simulink model "Friction_simulation"  (R2017b)
settings: Solver=FixedStepAuto  StartTime=0.0  StopTime=24  FixedStep=0.0005  MaxStep=0.0005  MinStep=0.0005  RelTol=1e-3
settings Model: Creator=zkt  LastModifiedBy=zkt

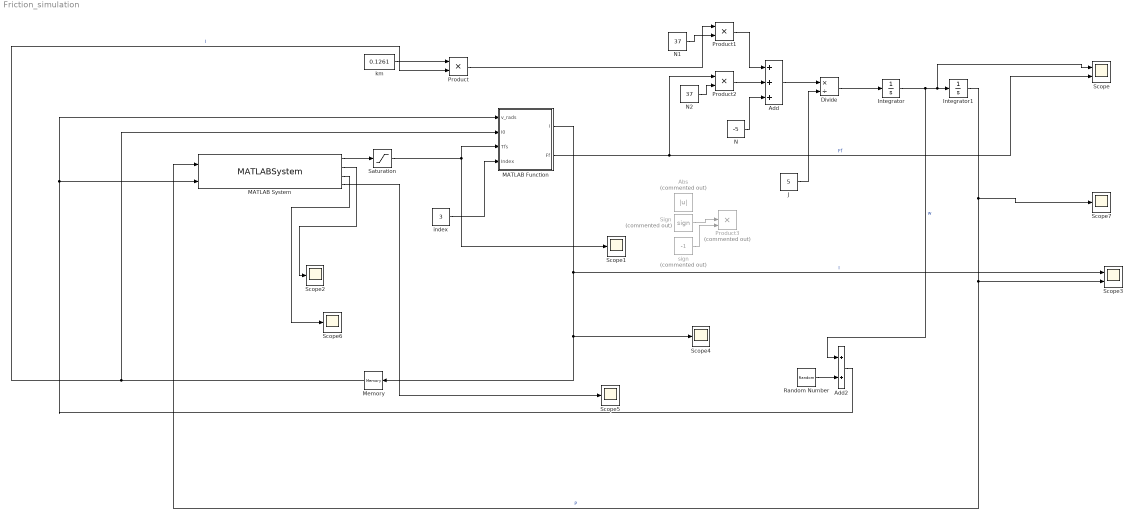
== system Friction_simulation ==
  Abs : Abs  Commented=on
  Add : Sum  Inputs=+++
  Add2 : Sum
  Divide : Product  Inputs=*/
  Integrator : Integrator
  Integrator1 : Integrator
  J : Constant  Value=5  OutDataTypeStr=double
  MATLAB Function : MATLAB Function  TreatAsAtomicUnit=on
  MATLAB System : MATLABSystem  System=Friction_simulation_control  SimulateUsing=Code generation
      mask Type: Friction_simulation_control
      mask Display:
      | disp('Friction_simulation_control');
      | port_label('input',1,'actuator_position');
      | port_label('input',2,'actuator_velocity');
      | port_label('output',1,'target_torque');
      | port_label('output',2,'random_w');
      | port_label('output',3,'random_I');
      | port_label('output',4,'simu_step');
  Memory : Memory
  N : Constant  Value=-5  OutDataTypeStr=double
  N1 : Constant  Value=37  OutDataTypeStr=double
  N2 : Constant  Value=37  OutDataTypeStr=double
  Product : Product
  Product1 : Product
  Product2 : Product
  Product3 : Product  Commented=on  Inputs=3
  Random Number : RandomNumber  Variance=0.01  SampleTime=0.0005
  Saturation : Saturate  UpperLimit=100  LowerLimit=-100
  Scope : Scope  NumInputPorts=2
  Scope{1..2,4..7} (6 alike) : Scope
  Scope3 : Scope  NumInputPorts=2
  Sign : Signum  Commented=on
  "index " : Constant  Value=3  OutDataTypeStr=int16
  km : Constant  Value=0.1261  OutDataTypeStr=double
  sign : Constant  Commented=on  Value=-1  OutDataTypeStr=double
  wires:
  km/1 -> Product/1
  Add/1 -> Divide/1
  Product/1 -> Product1/1
  "index "/1 -> MATLAB Function/4(Index)
  MATLAB Function/1(I) -> Memory/1, Scope4/1, Scope3/1  "I"
  J/1 -> Divide/2
  Divide/1 -> Integrator/1
  MATLAB System/2 -> Scope2/1
  N/1 -> Add/3
  MATLAB System/1 -> Saturation/1
  N1/1 -> Product1/2
  Product1/1 -> Add/1
  N2/1 -> Product2/2
  Product2/1 -> Add/2
  Integrator1/1 -> Scope7/1, Scope3/2, MATLAB System/1  "P"
  Saturation/1 -> MATLAB Function/3(Tfs), Scope1/1
  MATLAB System/4 -> Scope5/1
  MATLAB Function/2(Ff) -> Product2/1, Scope/2  "Ff"
  Sign/1 -> Product3/2
  sign/1 -> Product3/3
  MATLAB System/3 -> Scope6/1
  Random Number/1 -> Add2/2
  Integrator/1 -> Add2/1, Scope/1, Integrator1/1  "w"
  Memory/1 -> MATLAB Function/2(I0), Product/2  "I"
  Add2/1 -> MATLAB System/2, MATLAB Function/1(v_rads)

== matlab function Friction_simulation/MATLAB Function ==
  data: v_rads input; I output; I0 input; Tfs input; Index input; Ff output
function [I,Ff] = GetCurrent(v_rads,I0,Tfs,Index) %v:rad/s I:A %Tfs:NM output_torque 
    if Index ==3 || Index ==4   %三维模型
%         sigmoid_zoom = 2000;
        Km = 2.9/23;  %0.1261
        N=37; %减速比
        Te=I0*Km; %Te电扭矩 
%         v_rads_sign_current = sign(I0)*abs(v_rads);
        if v_rads >0 
            Ff = f_PO(v_rads,Te,Index);
        else
            Ff = f_NE(v_rads,Te,Index);
        end      
%         Ff = Ff*0.5;
        I=(Tfs-N*Ff)/(N*Km);
    elseif Index == 1    %旧模型
%         start_average =  1.39;
        Km1 = 2.9/23;
        N1=50;
        Te=I0*Km1; %Te电扭矩
%         v_rads_sign_current = sign(I0)*abs(v_rads);
        if v_rads > 0    
            Ff = f_PO_xiebo(v_rads,Te,Index);
        else 
            Ff = f_NE_xiebo(v_rads,Te,Index);
        end
%         Ff = Ff*0.5;
        I=(Tfs-N1*Ff)/(N1*Km1);
    else
        Ff =0;
        I= 0;
    end
end


function [z]= f_PO_xiebo(x,y,Index)
    ac = -0.5709;    
    as = -0.3521;  
    fc = 0.1078 ;
    fs = 0.1346; %adjust
    sigma = 0.009376;
    vs = 0.08399;
    z = -(fc+ac*y)-(fs+as*y-fc-ac*y)*exp(-x/vs)-sigma*x;
end
function [z]= f_NE_xiebo(x,y,Index)
    ac = -0.5873;    
    as = -0.332;  
    fc = 0.1144;
    fs = 0.1387; %adjust
    sigma =  0.0108;
    vs = 0.09723;
    z = fc-ac*y+(fs-as*y-fc+ac*y)*exp(x/vs)-sigma*x;
end
function [z]= f_PO(x,y,Index) 
%result
%        ac 常系数，表征电扭矩对库伦摩擦力矩的影响
%        as 常系数，表征电扭矩对静摩擦力矩的影响
%        fc 库伦摩擦力矩常数项
%        fs 静摩擦力矩常数项
%        sigma 粘滞摩擦系数
%        vs 临界Stribeck速度
%        x 速度rad/s
%        y 电扭矩NM=I*km
%        km=0.1261
% %PO:z1=f(x1,y1)
% General model:
%      f(x,y) = -(fc+ac*y)-(fs+as*y-fc-ac*y)*exp(-x/vs)-sigma*x
% Coefficients (with 95% confidence bounds):
%        ac =      0.1282  (0.1255, 0.131)
%        as =     0.08165  (0.06208, 0.1012)
%        fc =      0.1958  (0.1925, 0.1992)
%        fs =      0.3001  (0.2872, 0.313)
%        sigma =     0.02891  (0.02746, 0.03036)
%        vs =      0.1855  (0.1517, 0.2194)
%%%%%%%%%%%%%%%%%%%get average%%%%%%%%%%%%%%%%%%%%%
    ac = 0.1348;    
    as = 0.106975;  
    fc = 0.18785;
    if Index == 3
        fs = 0.289; %adjust
    elseif Index == 4
        fs = 0.189;
    else
        fs = 0.289;
    end 
    sigma = 0.02857;
    vs = 0.20095;
    z = -(fc+ac*y)-(fs+as*y-fc-ac*y)*exp(-x/vs)-sigma*x;
end

function [z]= f_NE(x,y,Index)
    ac = 0.1348;    
    as = 0.106975;  
    fc = 0.18785;
    if Index == 3
        fs = 0.289; %adjust
    elseif Index == 4
        fs = 0.189;
    else
        fs = 0.289;
    end 
    sigma = 0.02857;
    vs = 0.20095;
    z = fc-ac*y+(fs-as*y-fc+ac*y)*exp(x/vs)-sigma*x;
end
%NE:z2=f(x2,y2)
% General model:
%      f(x,y) = fc-ac*y+(fs-as*y-fc+ac*y)*exp(x/vs)-sigma*x
% Coefficients (with 95% confidence bounds):
%        ac =      0.1414  (0.1384, 0.1444)
%        as =      0.1323  (0.1138, 0.1509)
%        fc =      0.1799  (0.1759, 0.1839)
%        fs =      0.2584  (0.2458, 0.2709)
%        sigma =     0.02823  (0.02652, 0.02995)
%        vs =      0.2164  (0.1613, 0.2715)
